simulink model "SingleCylinderTest"  (R2014a)
settings: Solver=ode3  SolverMode=SingleTasking  StartTime=0.0  StopTime=5000.0  RelTol=1e-3
libraries: arduinolib x3
settings Model: ExtModeTrigDuration=2  Creator=beaverl  LastModifiedBy=beaverl
settings OptimizationCC: OptimizeModelRefInitCode=on  LifeSpan=1
settings DebuggingCC: UnderspecifiedInitializationDetection=Classic  SolverPrmCheckMsg=none
settings HardwareCC: ProdBitPerInt=16  ProdBitPerPointer=8  ProdIntDivRoundTo=Zero  ProdEndianess=LittleEndian  ProdWordSize=8  ProdHWDeviceType=Atmel->AVR
settings RTWCC: SystemTargetFile=realtime.tlc  GenerateMakefile=off  TemplateMakefile=realtime.tmf  Description=Run on Target Hardware  RTWVerbose=off  ProcessScript=realtime_make_rtw_hook
settings STFCustomTargetCC: TargetLibSuffix=.a  GenerateSampleERTMain=on  ConcurrentExecutionCompliant=off  GeneratePreprocessorConditionals=Use local settings  ERTCustomFileBanners=on  SupportNonInlinedSFcns=off  SupportVariableSizeSignals=on  MATLABClassNameForMDSCustomization=Simulink.SoftwareTarget.ERTCustomization  GRTInterface=off  SystemTargetFile=realtime.tlc
settings ERTTargetCC: CombineOutputUpdateFcns=off  SupportContinuousTime=on  SupportVariableSizeSignals=on  ExtModeTransport=3  ExtModeMexFile=ext_serial_win32_comm  ExtModeMexArgs=0 1 9600  ERTSrcFileBannerTemplate=realtime_code_template.cgt  ERTHdrFileBannerTemplate=realtime_code_template.cgt  ERTDataSrcFileTemplate=realtime_code_template.cgt  ERTDataHdrFileTemplate=realtime_code_template.cgt  ERTCustomFileTemplate=realtime_file_process.tlc

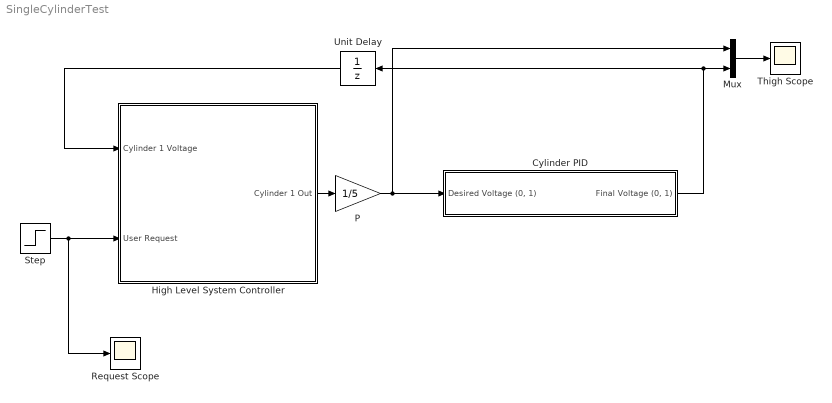
== system SingleCylinderTest ==
  Cylinder PID : Subsystem
  High Level System Controller : Subsystem
  Mux : Mux  Inputs=2
  P : Gain  Gain=1/5
  Request Scope : Scope
      settings: TimeRange=1  YMin=0.95  YMax=1.05
  Step : Step  Time=0  SampleTime=0.01
  Thigh Scope : Scope
      settings: TimeRange=1  YMin=1.88  YMax=2
  Unit Delay : UnitDelay  SampleTime=-1
  wires:
  High Level System Controller/1(Cylinder 1 Out) -> P/1
  Mux/1 -> Thigh Scope/1
  Unit Delay/1 -> High Level System Controller/1(Cylinder 1 Voltage)
  Step/1 -> Request Scope/1, High Level System Controller/2(User Request)
  P/1 -> Mux/1, Cylinder PID/1("Desired Voltage (0, 1)")
  Cylinder PID/1("Final Voltage (0, 1)") -> Unit Delay/1, Mux/2

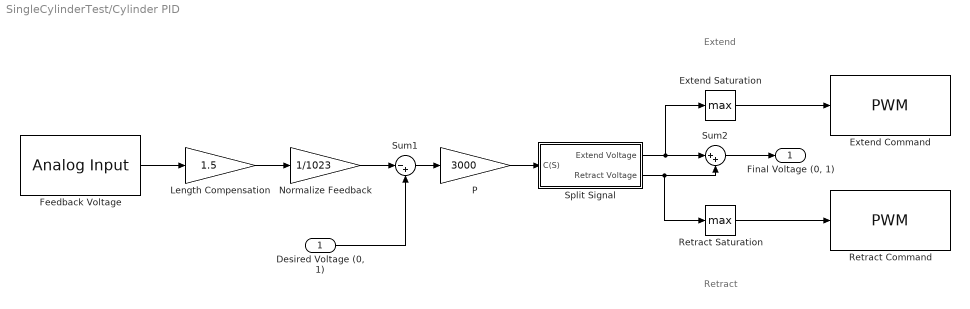
== system SingleCylinderTest/Cylinder PID ==
  note: Retract
  note: Extend
  "Desired Voltage (0, 1)" : Inport
  Extend Command : arduinolib/PWM  pinNumber=5
  Extend Saturation : MinMax  Function=max  OutMin=[0]  OutMax=[255]  OutDataTypeStr=int16  SaturateOnIntegerOverflow=on
  Feedback Voltage : arduinolib/Analog Input  pinNumber=2  sampleTime=-1
  Length Compensation : Gain  Gain=1.5
  Normalize Feedback : Gain  Gain=1/1023
  P : Gain  Gain=3000
  Retract Command : arduinolib/PWM  pinNumber=7
  Retract Saturation : MinMax  Function=max  OutMin=[0]  OutMax=[255]  OutDataTypeStr=int16  SaturateOnIntegerOverflow=on
  Split Signal : Subsystem
  Sum1 : Sum  Inputs=|-+
  Sum2 : Sum  Inputs=|++
  "Final Voltage (0, 1)" : Outport
  wires:
  Sum1/1 -> P/1
  Split Signal/1(Extend Voltage) -> Extend Saturation/1, Sum2/1
  Sum2/1 -> "Final Voltage (0, 1)"/1
  Feedback Voltage/1 -> Length Compensation/1
  Normalize Feedback/1 -> Sum1/1
  Split Signal/2(Retract Voltage) -> Retract Saturation/1, Sum2/2
  Extend Saturation/1 -> Extend Command/1
  Retract Saturation/1 -> Retract Command/1
  P/1 -> Split Signal/1(C(S))
  "Desired Voltage (0, 1)"/1 -> Sum1/2
  Length Compensation/1 -> Normalize Feedback/1

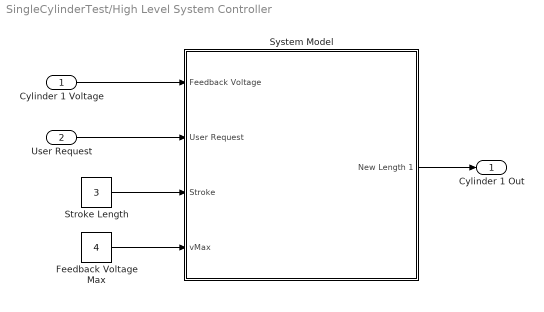
== system SingleCylinderTest/High Level System Controller ==
  Cylinder 1 Voltage : Inport  OutDataTypeStr=double
  User Request : Inport  Port=2
  Feedback Voltage Max : Constant  Value=4
  Stroke Length : Constant  Value=3
  System Model : Subsystem
  Cylinder 1 Out : Outport
  wires:
  Cylinder 1 Voltage/1 -> System Model/1(Feedback Voltage)
  Stroke Length/1 -> System Model/3(Stroke)
  Feedback Voltage Max/1 -> System Model/4(vMax)
  User Request/1 -> System Model/2(User Request)
  System Model/1(New Length 1) -> Cylinder 1 Out/1

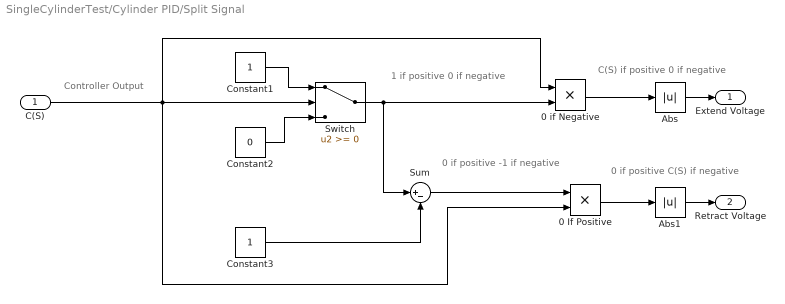
== system SingleCylinderTest/Cylinder PID/Split Signal ==
  note: Controller Output
  note: 0 if positive
      | C(S) if negative
  note: C(S) if positive
      | 0 if negative
  note: 0 if positive
      | -1 if negative
  note: 1 if positive
      | 0 if negative
  C(S) : Inport
  0 If Positive : Product
  0 if Negative : Product
  Abs : Abs
  Abs1 : Abs
  Constant1 : Constant
  Constant2 : Constant  Value=0
  Constant3 : Constant
  Sum : Sum  Inputs=|+-
  Switch : Switch
  Extend Voltage : Outport
  Retract Voltage : Outport  Port=2
  wires:
  Constant1/1 -> Switch/1
  Constant2/1 -> Switch/3
  Switch/1 -> 0 if Negative/2, Sum/1
  Constant3/1 -> Sum/2
  0 If Positive/1 -> Abs1/1
  C(S)/1 -> 0 If Positive/2, 0 if Negative/1, Switch/2
  Sum/1 -> 0 If Positive/1
  0 if Negative/1 -> Abs/1
  Abs/1 -> Extend Voltage/1
  Abs1/1 -> Retract Voltage/1

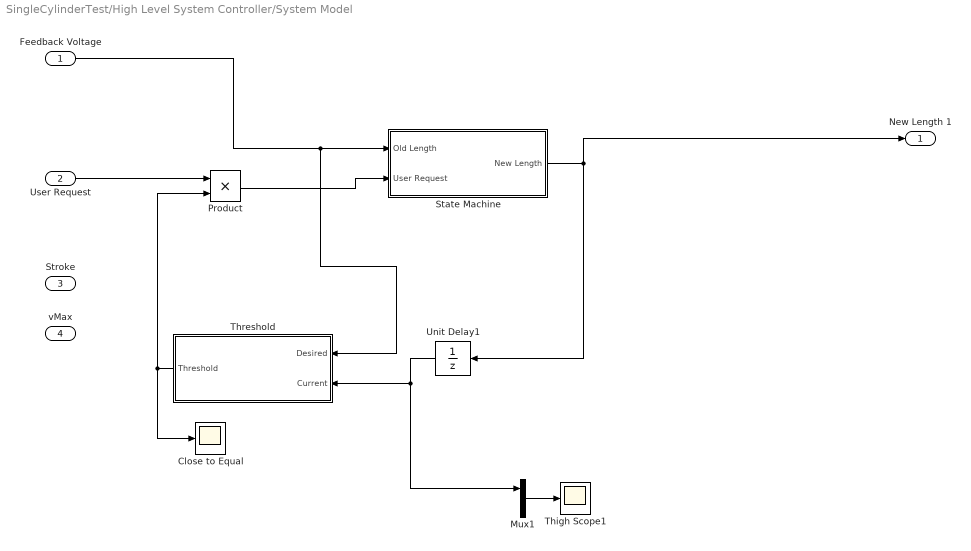
== system SingleCylinderTest/High Level System Controller/System Model ==
  Feedback Voltage : Inport
  User Request : Inport  Port=2
  Stroke : Inport  Port=3
  vMax : Inport  Port=4
  Close to Equal : Scope
      settings: TimeRange=1  YMin=2.53334  YMax=2.8  SaveName=ScopeData5
  Mux1 : Mux  Inputs=2
  Product : Product
  State Machine : Subsystem
  Thigh Scope1 : Scope
      settings: TimeRange=1  YMin=2.53334  YMax=2.8  SaveName=ScopeData4
  Threshold : Subsystem
  Unit Delay1 : UnitDelay  SampleTime=-1
  New Length 1 : Outport  OutDataTypeStr=double
  wires:
  State Machine/1(New Length) -> New Length 1/1, Unit Delay1/1
  Unit Delay1/1 -> Threshold/2(Current), Mux1/1
  Mux1/1 -> Thigh Scope1/1
  Threshold/1(Threshold) -> Close to Equal/1, Product/2
  Feedback Voltage/1 -> Threshold/1(Desired), State Machine/1(Old Length)
  User Request/1 -> Product/1
  Product/1 -> State Machine/2(User Request)

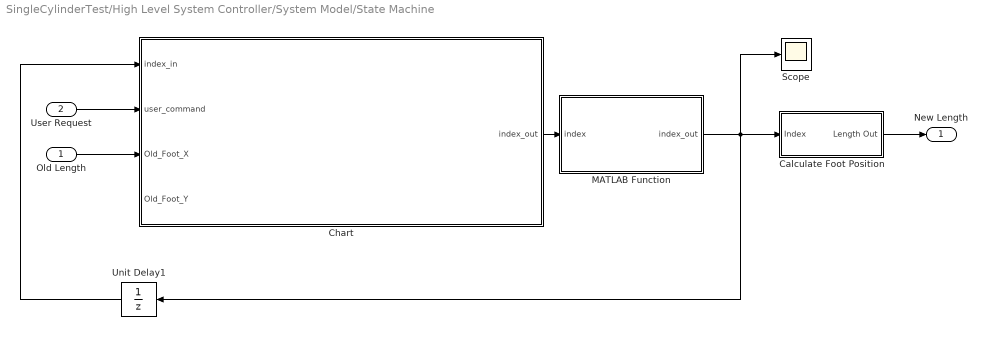
== system SingleCylinderTest/High Level System Controller/System Model/State Machine ==
  Old Length : Inport
  User Request : Inport  Port=2
  Calculate Foot Position : Subsystem
  Chart : Stateflow chart  TreatAsAtomicUnit=on
  MATLAB Function : MATLAB Function  TreatAsAtomicUnit=on
  Scope : Scope
      settings: SaveName=ScopeData2
  Unit Delay1 : UnitDelay  SampleTime=-1
  New Length : Outport
  wires:
  User Request/1 -> Chart/2(user_command)
  Calculate Foot Position/1(Length Out) -> New Length/1
  Old Length/1 -> Chart/3(Old_Foot_X)
  Unit Delay1/1 -> Chart/1(index_in)
  Chart/1(index_out) -> MATLAB Function/1(index)
  MATLAB Function/1(index_out) -> Unit Delay1/1, Scope/1, Calculate Foot Position/1(Index)

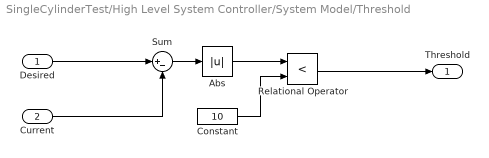
== system SingleCylinderTest/High Level System Controller/System Model/Threshold ==
  Desired : Inport
  Current : Inport  Port=2
  Abs : Abs
  Constant : Constant  Value=10
  Relational Operator : RelationalOperator  Operator=<  OutDataTypeStr=boolean
  Sum : Sum  Inputs=|+-
  Threshold : Outport
  wires:
  Desired/1 -> Sum/1
  Current/1 -> Sum/2
  Sum/1 -> Abs/1
  Constant/1 -> Relational Operator/2
  Relational Operator/1 -> Threshold/1
  Abs/1 -> Relational Operator/1

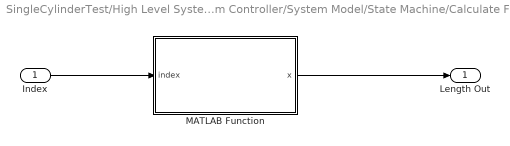
== system SingleCylinderTest/High Level System Controller/System Model/State Machine/Calculate Foot Position ==
  Index : Inport
  MATLAB Function : MATLAB Function  TreatAsAtomicUnit=on
  Length Out : Outport
  wires:
  MATLAB Function/1(x) -> Length Out/1
  Index/1 -> MATLAB Function/1(index)

== matlab function SingleCylinderTest/High Level System Controller/System Model/State Machine/Calculate Foot Position/MATLAB Function ==
  data: x output; index input
function x  = LookupTable(index)
%#codegen
indexTemp = index;
if(index < 1)
    indexTemp = 1;
elseif(index > 6)
    indexTemp = 6;
end;
Array = [1:4, 3:-1:2]; %divide by 5 to normalize

x = Array(indexTemp);

== stateflow chart SingleCylinderTest/High Level System Controller/System Model/State Machine/Chart ==
  state Idle
    entry: index_out = index_in;
  state Reverse
    entry: index_out = index_in - 1;
    during: index_out = index_in-1;
  state Forward
    entry: index_out = index_in + 1;
    during: index_out = index_in + 1;
  Reverse -> Idle : [user_command ~= -1]
  (default) -> Idle
  Idle -> Forward [order 1] : [user_command == 1]
  Forward -> Idle : [user_command ~= 1]
  Idle -> Reverse [order 2] : [user_command == -1]
  data: index_in input; user_command input; index_out output; Old_Foot_X input; Old_Foot_Y input

== matlab function SingleCylinderTest/High Level System Controller/System Model/State Machine/MATLAB Function ==
  data: index_out output; index input
function index_out = ClampIndex(index)
%#codegen
index_out = index;
if index > 6
    index_out = 1;
end
if index < 1
    index_out = 6;
end
